simulink model "TP1P08"  (R2017a)
settings: Solver=VariableStepAuto  StartTime=0.0  StopTime=10.0  RelTol=1e-3
values from neighbouring files (symbols this model uses):
  g = 9.81    [calcul_K.m]
undefined symbols (not defined in the file or in its folder): alpha0, l
libraries: simulink x1
settings Model: Creator=rxambili  LastModifiedBy=rxambili

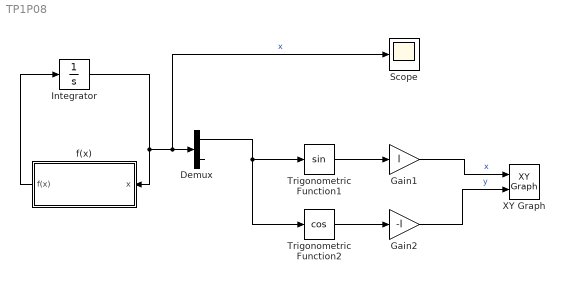
== system TP1P08 ==
  Demux : Demux  Outputs=2
  Gain1 : Gain  Gain=l
  Gain2 : Gain  Gain=-l
  Integrator : Integrator  InitialCondition=[ alpha0 0]
  Scope : Scope
  Trigonometric Function1 : Trigonometry
  Trigonometric Function2 : Trigonometry  Operator=cos
  XY Graph : simulink/Sinks/XY Graph  xmin=-2  xmax=2  ymin=-2  ymax=2  st=-1
  f(x) : Subsystem
  wires:
  f(x)/1(f(x)) -> Integrator/1
  Trigonometric Function2/1 -> Gain2/1
  Gain1/1 -> XY Graph/1  "x"
  Gain2/1 -> XY Graph/2  "y"
  Integrator/1 -> Scope/1, Demux/1, f(x)/1(x)  "x"
  Trigonometric Function1/1 -> Gain1/1
  Demux/2 -> ?
  Demux/1 -> Trigonometric Function2/1, Trigonometric Function1/1

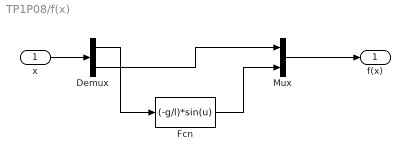
== system TP1P08/f(x) ==
  x : Inport
  Demux : Demux  Outputs=2
  Fcn : Fcn  Expr=(-g/l)*sin(u)
  Mux : Mux  Inputs=2
  f(x) : Outport
  wires:
  x/1 -> Demux/1
  Mux/1 -> f(x)/1
  Demux/1 -> Fcn/1
  Demux/2 -> Mux/1
  Fcn/1 -> Mux/2
